simulink model "STM"  (R2023b)
settings: Solver=FixedStepAuto  StartTime=0.0  StopTime=dt  FixedStep=dt  RelTol=1e-3
undefined symbols (not defined in the file): a, bias_acc, bias_clock, bias_gyro, drift_clock, q_m, v_b, v_m, w, x_b, x_m
libraries: nav_lib x2
settings Model: Creator=brent  LastModifiedBy=brent

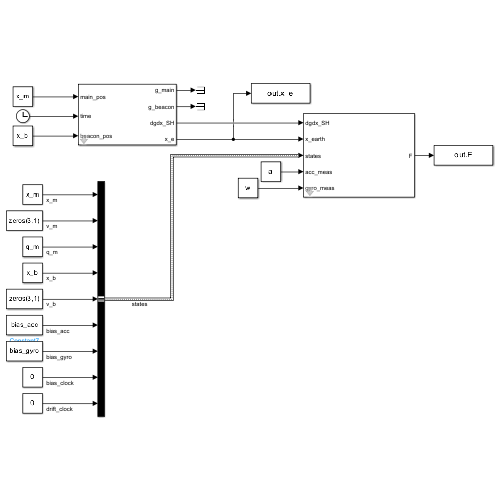
[thumbnail: Simulink's stored preview of the top-level diagram]
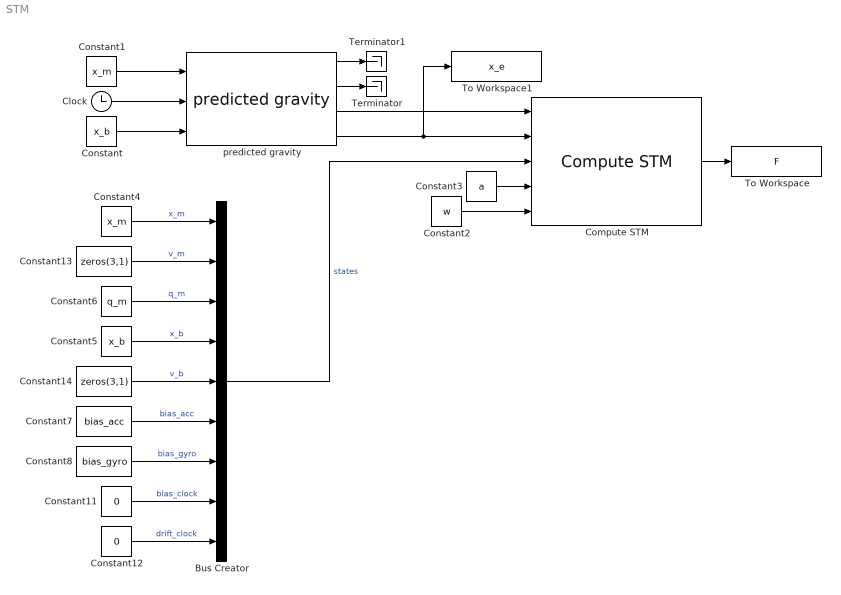
== system STM ==
  Bus Creator : BusCreator  Inputs=x_m,v_m,q_m,x_b,v_b,bias_acc,bias_gyro,bias_clock,drift_clock  OutDataTypeStr=Bus: statesBus  NonVirtualBus=on
  Clock : Clock
  Compute STM : nav_lib/Compute STM  dt=dt  mu_e=Propagation.Earth.mu.value  mu_m=Propagation.Moon.mu.value
      settings: SourceProductName=Navigation library
  Constant : Constant  Value=x_b
  Constant1 : Constant  Value=x_m
  Constant11 : Constant  Value=0
  Constant12 : Constant  Value=0
  Constant13 : Constant  Value=zeros(3,1)
  Constant14 : Constant  Value=zeros(3,1)
  Constant2 : Constant  Value=w
  Constant3 : Constant  Value=a
  Constant4 : Constant  Value=x_m
  Constant5 : Constant  Value=x_b
  Constant6 : Constant  Value=q_m
  Constant7 : Constant  Value=bias_acc
  Constant8 : Constant  Value=bias_gyro
  Terminator : Terminator
  Terminator1 : Terminator
  To Workspace : ToWorkspace  VariableName=F  SampleTime=-1
  To Workspace1 : ToWorkspace  VariableName=x_e  SampleTime=-1
  predicted gravity : nav_lib/predicted gravity  date=StartDate  Earth=Propagation.Earth  Moon=Propagation.Moon
      settings: SourceProductName=Navigation library
  wires:
  predicted gravity/3 -> Compute STM/1
  predicted gravity/4 -> To Workspace1/1, Compute STM/2
  predicted gravity/2 -> Terminator/1
  predicted gravity/1 -> Terminator1/1
  Clock/1 -> predicted gravity/2
  Constant/1 -> predicted gravity/3
  Constant1/1 -> predicted gravity/1
  Constant3/1 -> Compute STM/4
  Constant2/1 -> Compute STM/5
  Constant4/1 -> Bus Creator/1  "x_m"
  Bus Creator/1 -> Compute STM/3  "states"
  Compute STM/1 -> To Workspace/1
  Constant6/1 -> Bus Creator/3  "q_m"
  Constant11/1 -> Bus Creator/8  "bias_clock"
  Constant12/1 -> Bus Creator/9  "drift_clock"
  Constant13/1 -> Bus Creator/2  "v_m"
  Constant5/1 -> Bus Creator/4  "x_b"
  Constant14/1 -> Bus Creator/5  "v_b"
  Constant7/1 -> Bus Creator/6  "bias_acc"
  Constant8/1 -> Bus Creator/7  "bias_gyro"
